simulink model "H8_HEMS_comparacionNL_Lineal"  (R2022b)
settings: Solver=VariableStepAuto  StartTime=0.0  StopTime=0.1  RelTol=1e-3
values from neighbouring files (symbols this model uses):
  A3 = [0 0 0 757.149487996 0 278.788259426 0 0 0 0 197.196508939 0 ... (36 elements, 6x6)]    [matrices_linealizacion_hems.mat]
  B3 = [0 0 0 -0.0459993641186 -0.0505798680894 0.151580453785 0 0 0 -0.0459993641186 0.0505798680894 0.151580453785 ... (24 elements, 6x4)]    [matrices_linealizacion_hems.mat]
  C3 = [1 0 0 0 0 0 0 1 0 0 0 0 ... (36 elements, 6x6)]    [matrices_linealizacion_hems.mat]
  cg_nom = 0.567    [linealizacion_5gdl.m]    (also in linealizacion_HEMS.m)
  D3 = [0 0 0 0 0 0 0 0 0 0 0 0 ... (24 elements, 6x4)]    [matrices_linealizacion_hems.mat]
settings Model: Creator=USUARIO  LastModifiedBy=USUARIO

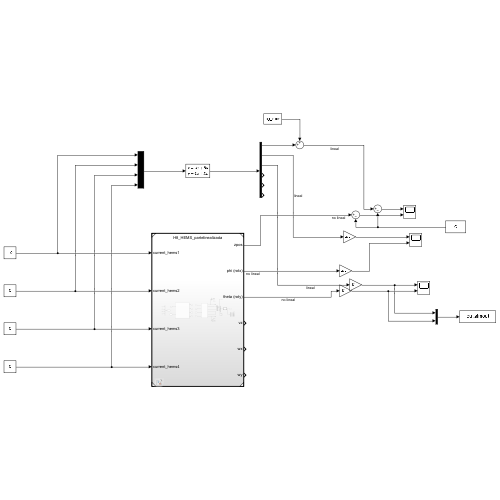
[thumbnail: Simulink's stored preview of the top-level diagram]
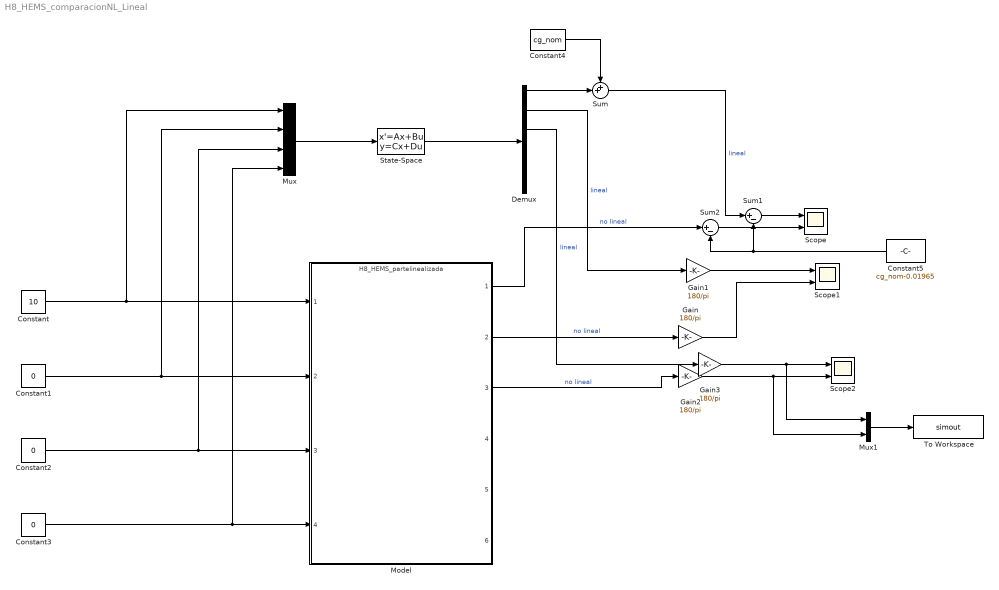
== system H8_HEMS_comparacionNL_Lineal ==
  Constant : Constant  Value=10
  Constant1 : Constant  Value=0
  Constant2 : Constant  Value=0
  Constant3 : Constant  Value=0
  Constant4 : Constant  Value=cg_nom
  Constant5 : Constant  Value=cg_nom-0.01965
  Demux : Demux  Outputs=6
  Gain{,1..3} (4 alike) : Gain  Gain=180/pi
  Model : ModelReference  ModelNameDialog=H8_HEMS_partelinealizada.slx  SimulationMode=Normal  ModelReferenceVersion=1.11
  Mux : Mux
  Mux1 : Mux  Inputs=2
  Scope : Scope  NumInputPorts=2
  Scope1 : Scope  NumInputPorts=2
  Scope2 : Scope  NumInputPorts=2
  State-Space : StateSpace  A=A3  B=B3  C=C3  D=D3  InitialCondition=[0 ,0 , 0.001 ,0 ,0 ,0]
  Sum : Sum  Inputs=++|
  Sum1 : Sum  Inputs=|+-
  Sum2 : Sum  Inputs=|+-
  To Workspace : ToWorkspace  VariableName=simout  SaveFormat=Timeseries  SampleTime=-1
  wires:
  Constant3/1 -> Mux/4, Model/4
  Constant2/1 -> Mux/3, Model/3
  Constant1/1 -> Mux/2, Model/2
  Constant/1 -> Mux/1, Model/1
  Mux/1 -> State-Space/1
  State-Space/1 -> Demux/1
  Sum/1 -> Sum1/1  "lineal"
  Model/1 -> Sum2/1  "no lineal"
  Demux/1 -> Sum/2
  Constant4/1 -> Sum/1
  Demux/2 -> Gain1/1  "lineal"
  Model/2 -> Gain/1  "no lineal"
  Demux/3 -> Gain3/1  "lineal"
  Model/3 -> Gain2/1  "no lineal"
  Sum1/1 -> Scope/1
  Constant5/1 -> Sum2/2, Sum1/2
  Sum2/1 -> Scope/2
  Gain1/1 -> Scope1/1
  Gain/1 -> Scope1/2
  Mux1/1 -> To Workspace/1
  Gain3/1 -> Mux1/1, Scope2/1
  Gain2/1 -> Mux1/2, Scope2/2
